simulink model "internet_movement"  (R2018b)
settings: Solver=VariableStepAuto  StartTime=0.0  StopTime=10.0  RelTol=1e-3
settings Model: Creator=Filipowicz_user1  LastModifiedBy=Filipowicz_user1

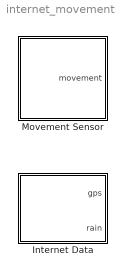
== system internet_movement ==
  Internet Data : Subsystem
  Movement Sensor : Subsystem

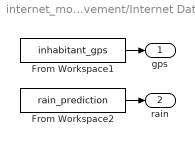
== system internet_movement/Internet Data ==
  From Workspace1 : FromWorkspace  VariableName=inhabitant_gps  SampleTime=0
  From Workspace2 : FromWorkspace  VariableName=rain_prediction  SampleTime=0
  gps : Outport
  rain : Outport  Port=2
  wires:
  From Workspace1/1 -> gps/1
  From Workspace2/1 -> rain/1

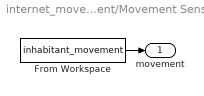
== system internet_movement/Movement Sensor ==
  From Workspace : FromWorkspace  VariableName=inhabitant_movement  SampleTime=0
  movement : Outport
  wires:
  From Workspace/1 -> movement/1
